simulink model "Simulink_1"  (R2017b)
settings: Solver=VariableStepAuto  StartTime=0.0  StopTime=10.0  RelTol=1e-3
undefined symbols (not defined in the file or in its folder): none, videoinput
libraries: imaqlib x1, visionsinks x1
settings Model: Creator=valakshe  LastModifiedBy=Vishwas Salunkhe

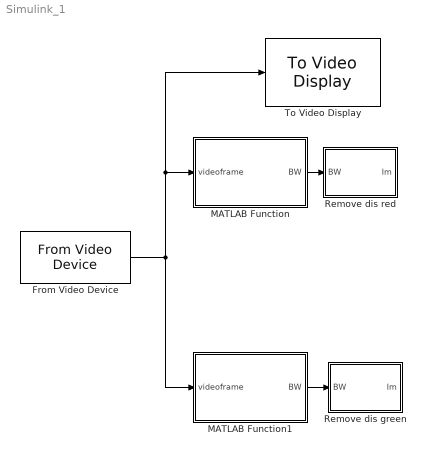
== system Simulink_1 ==
  From Video Device : imaqlib/From Video Device  DeviceMenu=winvideo 1 (HP Truevision HD)  Device=winvideo 1 (Integrated Camera)  ObjConstructor=videoinput('winvideo', 1)  VideoFormatMenu=MJPG_640x480  VideoFormat=MJPG_640x480  VideoSource=input1  ROIPosition=[0 0 480 640]  EnableHWTrigger=off  TriggerConfiguration=none/none  SampleTime=1/30  OutputPortsMode=One multidimensional signal  DataType=single  CanDoHWTrigger=no  ReturnedColorSpace=rgb  BlockHandle=25.0001  ROIWidth=640  ROIHeight=480  ROIColumn=0  ROIRow=0  EngXMLPath=E:\MATLAB\R2017b\toolbox\imaq\imaq\private  DevXMLPath=C:\ProgramData\MATLAB\SupportPackages\R2017b\toolbox\imaq\supportpackages\genericvideo\adaptor\win64  EngLibPath=E:\MATLAB\R2017b\toolbox\imaq\imaqblks\imaqmex\win64  ColorSpace=rgb  BayerSensorAlignment=grbg
      settings: SourceProductName=Image Acquisition Toolbox
  MATLAB Function : MATLAB Function  TreatAsAtomicUnit=on
  MATLAB Function1 : MATLAB Function  TreatAsAtomicUnit=on
  Remove dis green : MATLAB Function  TreatAsAtomicUnit=on
  Remove dis red : MATLAB Function  TreatAsAtomicUnit=on
  To Video Display : visionsinks/To Video Display  windowSizeMode=Normal  openAtMdlStart=on  fullScreen=off  videoWindowX=94  videoWindowY=166  saveWindowSize=off  videoWindowWidth=640  videoWindowHeight=480  inputColorFormat=RGB  inputType=Obsolete  imagePorts=One multidimensional signal  OutputDevice=On-screen video monitor  dataOrg=Column-major  isWindowOpen=off
      settings: SourceProductName=Computer Vision System Toolbox
  wires:
  MATLAB Function1/1(BW) -> Remove dis green/1(BW)
  From Video Device/1 -> MATLAB Function/1(videoframe), To Video Display/1, MATLAB Function1/1(videoframe)
  MATLAB Function/1(BW) -> Remove dis red/1(BW)

== matlab function Simulink_1/MATLAB Function1 ==
  data: videoframe input; BW output
function BW = fcn(videoframe)

    I = rgb2hsv(videoframe);

% Define thresholds for channel 1 based on histogram settings
    channel1Min = 0.476;
    channel1Max = 0.535;
    
    % Define thresholds for channel 2 based on histogram settings
    channel2Min = 0.486;
    channel2Max = 1.000;
    
    % Define thresholds for channel 3 based on histogram settings
    channel3Min = 0.257;
    channel3Max = 1.000;
    
    % Create mask based on chosen histogram thresholds
    BW = (I(:,:,1) >= channel1Min ) & (I(:,:,1) <= channel1Max) & ...
        (I(:,:,2) >= channel2Min ) & (I(:,:,2) <= channel2Max) & ...
        (I(:,:,3) >= channel3Min ) & (I(:,:,3) <= channel3Max);

== matlab function Simulink_1/MATLAB Function ==
  data: videoframe input; BW output
function BW = fcn(videoframe)

    I = rgb2hsv(videoframe);

    % Define thresholds for channel 1 based on histogram settings
    channel1Min = 0.925;
    channel1Max = 0.032;
    
    % Define thresholds for channel 2 based on histogram settings
    channel2Min = 0.127;
    channel2Max = 1.000;
    
    % Define thresholds for channel 3 based on histogram settings
    channel3Min = 0.349;
    channel3Max = 1.000;
    
    % Create mask based on chosen histogram thresholds
    BW = ( (I(:,:,1) >= channel1Min) | (I(:,:,1) <= channel1Max) ) & ...
        (I(:,:,2) >= channel2Min ) & (I(:,:,2) <= channel2Max) & ...
        (I(:,:,3) >= channel3Min ) & (I(:,:,3) <= channel3Max);

== matlab function Simulink_1/Remove dis green ==
  data: BW input; Im output
function Im = fcn(BW)

 diskElem = strel('disk',3);
 Im = imopen(BW,diskElem);

== matlab function Simulink_1/Remove dis red ==
  data: BW input; Im output
function Im = fcn(BW)

 diskElem = strel('disk',3);
 Im = imopen(BW,diskElem);
